simulink model "Model_Excel"  (R2020a)
settings: Solver=VariableStepAuto  StartTime=0.0  StopTime=inf  RelTol=1e-3
model workspace (MAT data in the model file):
  WinSize = 16
  fc_bandpass = [0.05 0.25]
undefined symbols (not defined in the file or in its folder): A1, A104210, D1, P104210, W1, W104210
libraries: gtecHighspeedLib x1, dspsigops x1, dspfdesign x1, dspstat3 x1
(part 2 of 2)

== system Model_Excel/zzz4 ==

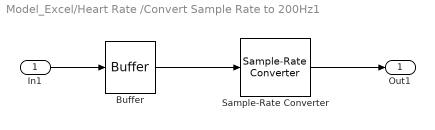
== system Model_Excel/Heart Rate /Convert Sample Rate to 200Hz1 ==
  In1 : Inport
  Buffer : Buffer  N=207
  Sample-Rate Converter : dspsigops/Sample-Rate Converter  InputSampleRate=512  OutputSampleRate=200  OutputRateTolerance=0.01  Bandwidth=198  StopbandAttenuation=60  SimulateUsing=Code generation
      settings: SourceProductBaseCode=DS
  Out1 : Outport
  wires:
  Buffer/1 -> Sample-Rate Converter/1
  Sample-Rate Converter/1 -> Out1/1
  In1/1 -> Buffer/1

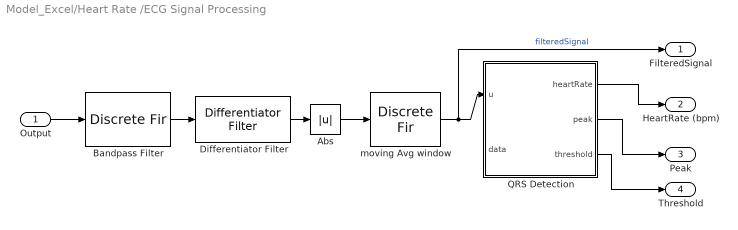
== system Model_Excel/Heart Rate /ECG Signal Processing ==
  Output : Inport
  Abs : Abs
  Bandpass Filter : DiscreteFir  DialogController=Simulink.DDGSource  Coefficients=fir1(256,fc_bandpass)  InputProcessing=Columns as channels (frame based)
  Differentiator Filter : dspfdesign/Differentiator Filter  DesignForMinimumOrder=off  FilterOrder=51  PassbandRipple=0.1  ScaleCoefficients=off  SimulateUsing=Interpreted execution  roundingMode=Floor  coeffsDataTypeStr=fixdt(1,16)
      settings: SourceProductBaseCode=DS
  QRS Detection : MATLAB Function  TreatAsAtomicUnit=on
  moving Avg window : DiscreteFir  DialogController=Simulink.DDGSource  Coefficients=ones(1, WinSize, 'single')/WinSize  InputProcessing=Columns as channels (frame based)
  FilteredSignal : Outport
  HeartRate (bpm) : Outport  Port=2
  Peak : Outport  Port=3
  Threshold : Outport  Port=4
  wires:
  Differentiator Filter/1 -> Abs/1
  QRS Detection/1(heartRate) -> HeartRate (bpm)/1
  Bandpass Filter/1 -> Differentiator Filter/1
  Abs/1 -> moving Avg window/1
  QRS Detection/3(threshold) -> Threshold/1
  QRS Detection/2(peak) -> Peak/1
  Output/1 -> Bandpass Filter/1
  moving Avg window/1 -> FilteredSignal/1, QRS Detection/1(u)  "filteredSignal"

== matlab function Model_Excel/MATLAB Function ==
  data: u input; y output
function y = fcn(u)
%#codegen

y = (u*10)+10;

== matlab function Model_Excel/Ratioo/multipul ch mean2 ==
  data: u input; Mean_Ratio_multipul_ch output
function Mean_Ratio_multipul_ch = EEG_Stress_Ratio(u)

   coder.extrinsic('pwelch');
   coder.extrinsic('table2array');
   sampling_rate = 512;
   psd = zeros(513,1);
   frequencies = zeros(513,1);
   
   %initialize an array to store the stress scores for each channel
   stress_scores = zeros(size(u, 2), 1);
   disp(size(u));
   
       for i = 1:size(u, 2)
            
           %extract for current channel
           channel_data = u(:, i);
            
           % Calculate the power spectral density (PSD) of the EEG data
           [psd, frequencies] = pwelch(channel_data, [], [], [], sampling_rate);


           % Calculate the relative power in the alpha frequency band (8-12 Hz)
           alpha_power = sum(psd(frequencies >= 8 & frequencies <= 12)) / sum(psd);

           % Calculate the relative power in the beta frequency band (12-30 Hz)
           beta_power = sum(psd(frequencies >= 12 & frequencies <= 30)) / sum(psd);

           % Calculate the alpha/beta ratio for the current channel
%            alpha_beta_ratio = beta_power / alpha_power ;
             alpha_beta_ratio = log(beta_power) - log(alpha_power) ;


            stress_scores(i) = alpha_beta_ratio;
            
       end
  
 
    Mean_Ratio_multipul_ch = mean(stress_scores);
end

== matlab function Model_Excel/Heart Rate /ECG Signal Processing/QRS Detection ==
  data: heartRate output size=81; peak output; u input; threshold output; data input
function [heartRate,peak,threshold]  = QRSDetection(u, data)
% Description:
%   QRS Dectector based on the band-pass filtered ECG signal.
%   The QRS detection rules reference the PIC based QRS detector
%   implemented by Patrick S. Hamilton in picqrs.c
%   from Open Source ECG Analysis (OSEA)
%   http://www.eplimited.com/confirmation.htm
%
% INPUT:
%  u : bandpass filtered and moving averaged ECG signal
%
% OUTPUTS:
%  heartRate: detected heart rate (beat per minute)
%  peak     : detected local peaks (mainly R peaks)
%  threshold: the detection threshold is calculated based on
%             the mean estiamtes of the average QRS peak and
%             the average noise peak.
%
% Detection Rules:
% Rule 1. Ignore all peaks that precede or follow larger peaks by less
%         than 196 ms (306bpm). The EC13 Standard specifies that the
%         QRS detector should accurately detect QRS complexes at rates
%         as high as 250 beats-per-minute (bpm), and should not report
%         heart rates lower than 250bpm when rates as high as 300bpm occur.
% Rule 2. If a peak occurs, check to see whether the raw signal
%         contained both positive and negative slopes. If yes, 
%           report a peak being found, otherwise, the peak 
%           represents a baselien shift.
% Rule 3. If the peak is larger than the detection threshold 
%           classify it as a QRS complex, otherwise classify 
%           it as noise.
% Rule 4. If no QRS has been detected within 1.5 R-to-R intervals, 
%         there was a peak that was larger than half the
%         detection threshold, and the peak followed the preceding
%         detection by at least 360ms, classify that peak as a QRS
%         complex.


    persistent FS QRSDelay
    if isempty(FS)
        FS = 200; % Hz, samples per second
        QRSDelay = zeros(size(u), 'like', u);
    end
    
    
    heartRate = uint16(zeros(size(u)));
    peak = zeros(size(u), 'like', u);    
    threshold = zeros(size(u), 'like', u);
    % Prevents detections of peaks smaller than 150 uV.
    MIN_PEAK_AMP = cast(7/2^12, 'like', u(1));

    for idx = 1:length(u) 
        % For a frame of input signal, process one sample at a time
        peak(idx) = findpeak(u(idx));

        if(peak(idx) < MIN_PEAK_AMP)
            peak(idx) = 0 ;
        end

        % returns adjusted peak
        [QRSDelay(idx), threshold(idx), peak(idx)] = qrs_det(peak(idx));
        if QRSDelay(idx) ~= 0
            % beat per min = samplesPerSec * 60sec/min / samples per beat_oneQRSDalay
            heartRate(idx) = int16(60 * FS / QRSDelay(idx));
        end

    end
end % function QRSDetection


function pk = findpeak(datum)
    % peak() takes a datum as input and returns a peak height
    % when the signal returns to half its peak height, or it has been
    % 95 ms since the peak height was detected.
    
    persistent maxPeak lastDatum timeSinceMax
    pk = cast(0,'like',datum);
    if isempty(maxPeak)
        maxPeak = cast(0,'like',datum);
        lastDatum = cast(0,'like',datum);
        timeSinceMax = uint16(0);
        return
    end
    
    if timeSinceMax > 0
        timeSinceMax(:) = timeSinceMax + 1;
    end
    
    if((datum > lastDatum) && (datum > maxPeak)) % rising slope
        maxPeak(:) = datum ;
        if(maxPeak > 2) % reset timeSinceMax 
            timeSinceMax(:) = 1 ;
        end
    elseif(datum < bitsra(maxPeak,1)) % middle of falling slope
        % Less than half the peak height
        pk(:) = maxPeak ;
        maxPeak(:) = 0 ;
        timeSinceMax(:) = 0 ;
    elseif(timeSinceMax > MS95)
        pk(:) = maxPeak ;
        maxPeak(:) = 0 ;
        timeSinceMax(:) = 0 ;
    end
    lastDatum = datum ;
end

function [QRSDelay,thisThreshold, pk] = qrs_det(pk)
    
    persistent count 
    persistent qpkcnt
    persistent lastQRSDelay
    persistent threshold
    persistent preBlankCnt
    persistent tempPeak
    persistent initMax
    persistent sbpeak
    persistent sbcount
        
    if isempty(lastQRSDelay)
        count = int16(0);
        qpkcnt = int16(0);
        lastQRSDelay = int16(0);
        % EC13: QRS detector should not detect QRS complexes with 
        %  amplitudes of less than 0.15mV and 1mV QRS complexes with width
        %  less than 10ms (6000bpm)
        threshold = cast(8/2^12, 'like', pk);
        tempPeak = cast(0, 'like', pk);
        initMax = cast(0, 'like', pk);
        preBlankCnt = int16(0);
        sbpeak = cast(0, 'like', pk);
        sbcount = int16(MS1650);
    end
    
    % there can only be one QRS complex in any 196ms (306bpm) window
    if (pk==0) && (preBlankCnt==0)
        pk(:) = 0;
    elseif (pk==0) && (preBlankCnt~=0)
        % if we have held onto a peak for 196ms, pass it on for eval
        preBlankCnt = preBlankCnt - 1;
        if (preBlankCnt == 0)
            pk(:) = tempPeak;
        else
            pk(:) = 0;
        end        
    elseif (pk~=0) && (preBlankCnt==0)
        % if there has been no peak for 196ms, save this one and start
        % counting
        tempPeak = pk;
        preBlankCnt = MS196;
        pk(:) = 0;
    else % (pk~=0) &&  (preBlankCnt~=0)
        % if we were holding a peak, but this one is bigger,
        % save it and start counting to 196ms again
        if (pk > tempPeak)
            tempPeak = pk;
            preBlankCnt = MS196;
            pk(:) = 0;
        else
            preBlankCnt = preBlankCnt - 1;
            if (preBlankCnt == 0)
                pk(:) = tempPeak;
            else
                pk(:) = 0;
            end
        end
    end
    
    count(:) = count + 1;
    
    % Initialize the QRS peak buffer with the first eight 
    % local maximum peaks detected
    if qpkcnt < 8
        if pk > 0
           UPDATEQ = true;
           threshold = updateQN(pk, UPDATEQ);
           qpkcnt = qpkcnt + 1;
           if pk > initMax 
               initMax = pk;
           end
           if qpkcnt == 8
               count(:) = 0;
           end
           
        end
        
    else % qpkcnt >= 8
        
        if pk > threshold
            UPDATEQ = true;
            threshold = updateQN(pk, UPDATEQ);
            lastQRSDelay(:) = count;
            count(:) = 0;
            sbpeak(:) = 0;
        elseif pk ~= 0
            % if peak is below threshold
            UPDATEQ = false;
            threshold = updateQN(pk, UPDATEQ);
            
            % If no QRS has been detected within 1.5 R-to-R intervals, 
            % there was a peak that was larger than half the 
            % detection threshold, and the peak followed the preceding 
            % detection by at least 360ms, classify that peak as a QRS 
            % complex
            
            % persistent sbpeak = 0; sbcount = MS1650
            if (count >= MS360) && (pk > sbpeak)
                sbpeak = pk;
                sbloc = count;
                threshold(:) = bitsra(threshold,1);
                
                if (count > sbcount) && (sbpeak > threshold)
                    sbcount = updateRR(sbloc);
                    lastQRSDelay(:) = count;
                    % threshold = threshold >> 1;
                    count(:) = 0;
                    sbpeak(:) = 0;
                end
            end
            
        end
    end
    QRSDelay = lastQRSDelay;
    thisThreshold = threshold;
end

%**************************************************************************
%  UpdateQN takes a new QRS or noise peak value and updates the
%  QRS or noise mean estimate and detection threshold.
%  Input :
%  x - new QRS peak or noise peak value
%  Qflag - true (update QRS mean estimate), 
%          false (update Noise mean estimate)
% **************************************************************************/
function det_thresh = updateQN(x, Qflag)
  persistent QSum
  persistent NSum
  persistent Qz Nz nQ nN

  if isempty(NSum)
      nQ = uint8(0);
      nN = uint8(0);
      Qz = zeros(8,1,'like',x);
      Nz = zeros(8,1,'like',x);
      QSum = cast(0, 'like', x);
      NSum = cast(0, 'like', x);
  end

  det_thresh = cast(0, 'like', x);
  if Qflag %&& x ~= cast(0,'like',x)
      Qz(nQ+1) = x;
      nQ = bitand(nQ+1,uint8(7));
      QSum(:) = sum(Qz);
  else
      Nz(nN+1) = x;
      nN = bitand(nN+1,uint8(7));
      NSum(:) = sum(Nz);
  end
  det_thresh(:) = QSum-NSum ;
  det_thresh(:) = NSum + bitsra(det_thresh,1) - bitsra(det_thresh,3);
  det_thresh(:) = bitsra(det_thresh, 3);
end

%**************************************************************************
%  UpdateRR takes a new RR value and updates the RR mean estimate
%*************************************************************************/
function sbcount = updateRR(x)
  persistent RRSum
  persistent zR 
  persistent nR

  if isempty(RRSum)
      nR = uint8(0);
      zR = cast(MS1000*ones(8,1, 'int16'),'like',x);
      RRSum = cast(bitsll(MS1000,3), 'like', x);
  end
  
  sbcount = cast(0, 'like', x);
  zR(nR+1) = x;
  nR = bitand(nR+1,uint8(7));
  RRSum(:) = sum(bitsra(zR,3));
  
  sbcount(:) = RRSum + bitsra(RRSum, 1); % = 1.5RRSum
  sbcount(:) = bitsra(sbcount, 3);
  sbcount(:) = sbcount + MS80; % WINDOW_WIDTH
end

function n = MS80
% The number of samples in 95 milli-seconds, where FS is the sample rate
    FS = 200;
    n = int16(80 * FS / 1000);
end

function n = MS95
% The number of samples in 95 milli-seconds, where FS is the sample rate
    FS = 200;
    n = int16(95 * FS / 1000);
end

function n = MS196
% The number of samples in 196 milli-seconds, where FS is the sample rate
    FS = 200;
    n = int16(196 * FS / 1000);
end

function n = MS360
% The number of samples in 360 milli-seconds, where FS is the sample rate
    FS = 200;
    n = int16(360 * FS / 1000);
end

function n = MS1000
% The number of samples in 1000 milli-seconds, where FS is the sample rate
    FS = 200;
    n = int16(1000 * FS / 1000);
end

function n = MS1650
% The number of samples in 1650 milli-seconds, where FS is the sample rate
    FS = 200;
    n = int16(1650 * FS / 1000);
end

== matlab function Model_Excel/Mental load alguritom HR ==
  data: u input; y output
function y = fcn(u)

y= probability_of_mental_load_HR(u);

end

== matlab function Model_Excel/Mental load alguritom EEG ==
  data: u input; y output
function y = fcn(u)

y= probability_of_metal_load_EEG(u);

end

== matlab function Model_Excel/MATLAB Function2 ==
  data: u input; y output
function y = fcn(u)
%#codegen

y = (u*10)+10;
